simulink model "mcb_hostmodel_dsPIC33A"  (R2025b)
settings: Solver=FixedStepDiscrete  StartTime=0.0  StopTime=inf  RelTol=1e-3  EnableMultiTasking=on
values from neighbouring files (symbols this model uses):
  Ts_serialOut = 500e-6    (= 0.0005)    [mchp_pmsm_foc_smo_dsPIC33_data.m]
undefined symbols (not defined in the file or in its folder): target
libraries: instrumentseriallib x3
settings Model: Creator=The MathWorks, Inc.  LastModifiedBy=I50990
settings SolverCC: AlgebraicLoopSolver=TrustRegion  MaxZcPerStep=1.0
settings DataIOCC: LimitDataPoints=on  SaveFormat=Array  ReturnWorkspaceOutputs=off
settings OptimizationCC: ReuseModelBlockBuffer=off  LifeSpan=1  EfficientTunableParamExpr=on
settings DebuggingCC: UnderspecifiedInitializationDetection=Classic  MergeDetectMultiDrivingBlocksExec=none  SolverPrmCheckMsg=warning  ParameterPrecisionLossMsg=none  UnconnectedInputMsg=warning  UnconnectedOutputMsg=warning  UnconnectedLineMsg=warning  AllowSymbolicDim=off  PregeneratedLibrarySubsystemCodeDiagnostic=none  SFUnexpectedBacktrackingDiag=warning  SFNoUnconditionalDefaultTransitionDiag=warning  SFExecutionAtInitializationDiag=none  ArithmeticOperatorsInVariantConditions=warning
settings HardwareCC: ProdBitPerPointer=32.0  ProdLargestAtomicFloat=None  ProdIntDivRoundTo=Undefined  ProdEndianess=Unspecified  ProdWordSize=32.0  ProdHWDeviceType=32-bit Generic
settings ModelReferenceCC: EnableRefExpFcnMdlSchedulingChecks=on  PropagateSignalLabelsOutOfModel=off
settings SFSimCC: SimUseLocalCustomCode=off  MATLABDynamicMemAlloc=off
settings RTWCC: SystemTargetFile=ert.tlc  TemplateMakefile=ert_default_tmf  GenerateReport=on  RTWUseLocalCustomCode=off  IncludeHyperlinkInReport=on  LaunchReport=on  GenerateTraceInfo=on  GenerateTraceReport=on  GenerateTraceReportSl=on  GenerateTraceReportSf=on  GenerateTraceReportEml=on  GPUComputeCapability=3.5  DLArmComputeVersion=19.05  Description=Real-Time Workshop Embedded Coder
settings CodeAppCC: IgnoreCustomStorageClasses=off  StateflowObjectComments=on  InternalIdentifier=Classic
settings ERTTargetCC: InlinedParameterPlacement=Hierarchical  ERTCustomFileTemplate=example_file_process.tlc  ConvertIfToSwitch=off  SuppressUnreachableDefaultCases=off  DynamicArrayContainerType=coder::array  MultiwordLength=2048.0  GenerateSampleERTMain=on
settings ConfigComp: CovMetricSettings=dw  CovSaveCumulativeToWorkspaceVar=on  CovSaveSingleToWorkspaceVar=on  CovExternalEMLEnable=off  CovSFcnEnable=off

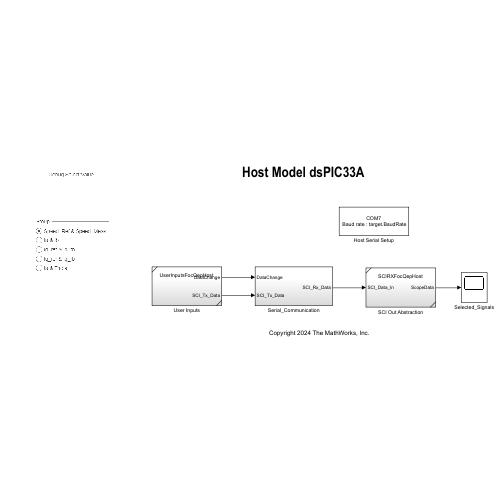
[thumbnail: Simulink's stored preview of the top-level diagram]
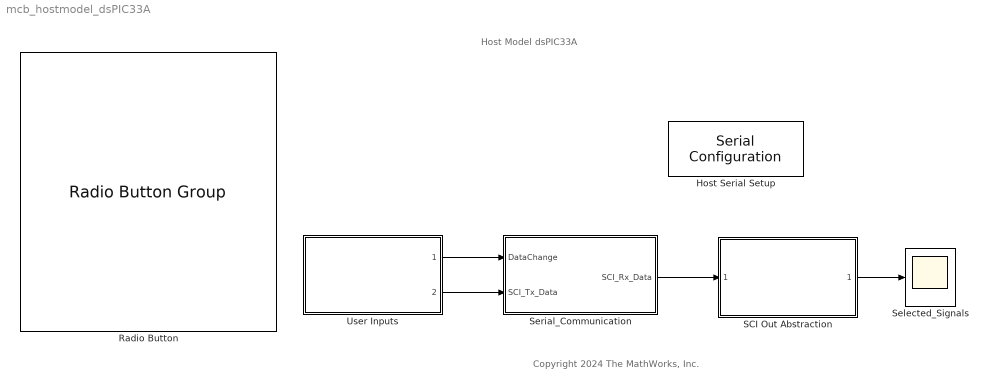
== system mcb_hostmodel_dsPIC33A ==
  note: Host Model dsPIC33A
  note: Copyright 2024 The MathWorks, Inc.
  Host Serial Setup : instrumentseriallib/Serial Configuration  Priority=-99  PortSel=target.comport  Port=target.comport  ComPort=target.comport  BaudRate=target.BaudRate  DataBits=8  Parity=none  StopBits=1  ByteOrder=little-endian  FlowControl=none  Timeout=2  SimulateUsing=Interpreted execution  BlockInModel=on  aMode=5
  Radio Button : RadioButtonGroup  SelectedLabel=Speed_Ref & Speed_Meas  ButtonGroupName=Group
  SCI Out Abstraction : Subsystem  ReferencedSubsystem=SCIRXFocQepHost
  Selected_Signals : Scope
      settings: TimeSpan=10  ActiveDisplayYMinimum=240.379264831543  ActiveDisplayYMaximum=1385.6375198364258  DataLoggingVariableName=Results_HW
  Serial_Communication : Subsystem
  User Inputs : Subsystem  ReferencedSubsystem=UserInputsFocQepHost
  wires:
  User Inputs/2 -> Serial_Communication/2(SCI_Tx_Data)
  User Inputs/1 -> Serial_Communication/1(DataChange)
  Serial_Communication/1(SCI_Rx_Data) -> SCI Out Abstraction/1
  SCI Out Abstraction/1 -> Selected_Signals/1

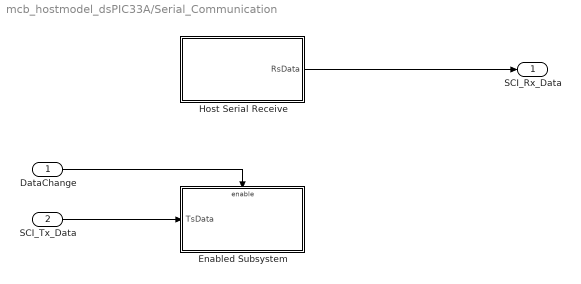
== system mcb_hostmodel_dsPIC33A/Serial_Communication ==
  DataChange : Inport
  SCI_Tx_Data : Inport  Port=2
  Enabled Subsystem : Subsystem  TreatAsAtomicUnit=on
  Host Serial Receive : Subsystem
  SCI_Rx_Data : Outport
  wires:
  DataChange/1 -> Enabled Subsystem/Enable
  SCI_Tx_Data/1 -> Enabled Subsystem/1(TsData)
  Host Serial Receive/1(RsData) -> SCI_Rx_Data/1

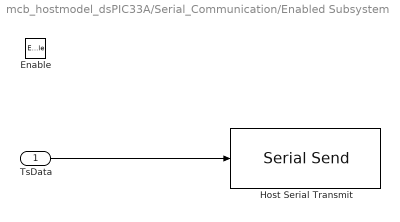
== system mcb_hostmodel_dsPIC33A/Serial_Communication/Enabled Subsystem ==
  TsData : Inport
  Enable : EnablePort
  Host Serial Transmit : instrumentseriallib/Serial Send  PortSel=target.comport  Port=target.comport  ComPort=target.comport  Header=[]  Terminator=<none>  CustomTerminator=[]  EnableBlockingMode=off  SimulateUsing=Interpreted execution  BlockInModel=on  aMode=5
  wires:
  TsData/1 -> Host Serial Transmit/1

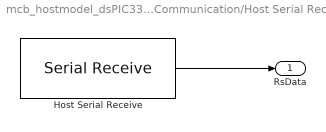
== system mcb_hostmodel_dsPIC33A/Serial_Communication/Host Serial Receive ==
  Host Serial Receive : instrumentseriallib/Serial Receive  PortSel=target.comport  Port=target.comport  ComPort=target.comport  DataType=single  SaveDataType=uint8  ToggleHeader=on  Header='S'  ToggleDataSize=on  DataSize=[target.frameSize 2]  ToggleTerminator=on  Terminator=Custom terminator  CustomTerminator='E'  InputFormat=Row major  EnableBlockingMode=on  ActionDataUnavailable=Output custom value  ActionWhenDataUnavailable=Output custom value  CustomValue=4  SampleTime=target.frameSize * Ts_serialOut  SimulateUsing=Interpreted execution  BlockInModel=on  aMode=5  LibraryInUse=instrumentlib
  RsData : Outport
  wires:
  Host Serial Receive/1 -> RsData/1
